simulink model "AAIver1"  (R2022a)
settings: Solver=VariableStepAuto  StartTime=0.0  StopTime=10.0  RelTol=1e-3
undefined symbols (not defined in the file): D0, D10, D11, D2, D3, D4, D8, D9, PTA0, PTA1, PTB23, PTB9, PTC16, PTC4, PTD0, PTD2
libraries: frdmk64flib x8
settings Model: Creator=Motz  LastModifiedBy=bmile

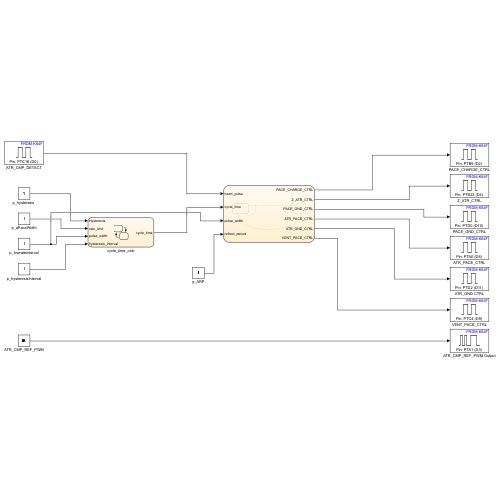
[thumbnail: Simulink's stored preview of the top-level diagram]
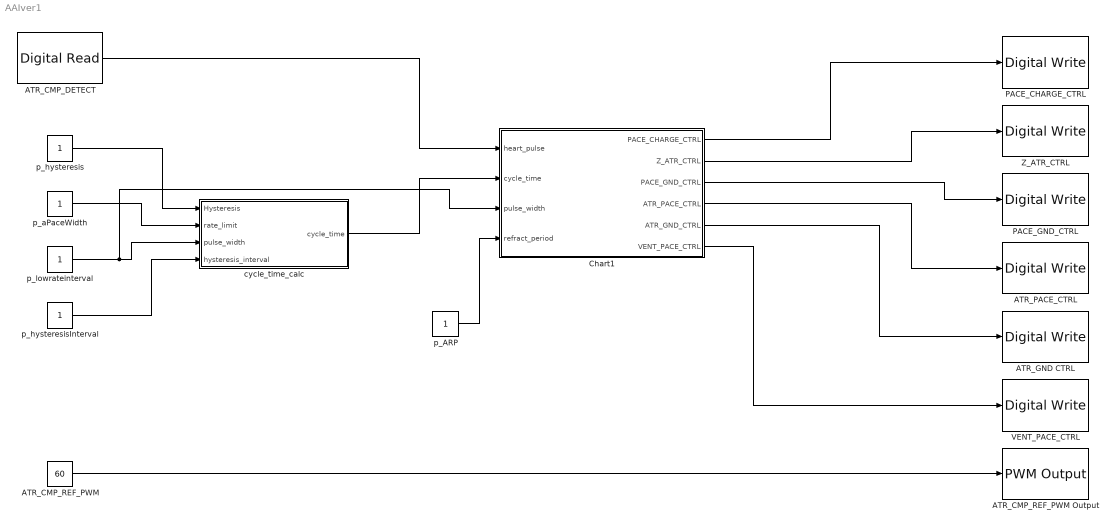
== system AAIver1 ==
  ATR_CMP_DETECT : frdmk64flib/Digital Read  Whichpin=PTC16 (D0)  SampleTime=-1
  ATR_CMP_REF_PWM : Constant  Value=60
  ATR_CMP_REF_PWM Output : frdmk64flib/PWM Output  Whichpin=PTA1 (D3)  InitialFrequency=2000  InitialDutyCycle=0
  ATR_GND CTRL : frdmk64flib/Digital Write  Whichpin=PTD2 (D11)
  ATR_PACE_CTRL : frdmk64flib/Digital Write  Whichpin=PTA0 (D8)
  Chart1 : Stateflow chart  TreatAsAtomicUnit=on
  PACE_CHARGE_CTRL : frdmk64flib/Digital Write  Whichpin=PTB9 (D2)
  PACE_GND_CTRL : frdmk64flib/Digital Write  Whichpin=PTD0 (D10)
  VENT_PACE_CTRL : frdmk64flib/Digital Write  Whichpin=PTC4 (D9)
  Z_ATR_CTRL : frdmk64flib/Digital Write  Whichpin=PTB23 (D4)
  cycle_time_calc : Stateflow chart  TreatAsAtomicUnit=on
      settings: PortSchema="{\"entries\":[{\"content\":{\"sides\":[{\"content\":{\"connectorIds\":[\"In1\",\"In2\",\"In4\",\"In3\"]},\"type\":\"ConnectorPlacement.EquallySpacedRectSide\",\"uuid\":\"0a7d0b3b-55bc-4c6a-8e46-ab8e8d3ba457\"},{\"content\":{\"connectorIds\":[\"Out1\"],\"side\":\"RIGHT\"},\"type\":\"ConnectorPlacement.EquallySpacedRectSide\",\"uuid\":\"eaa3c3bc-2449-459b-9c1e-a00ffc7b6bdb\"},{\"content\":{\"connectorIds\":[],\"side\":\"TOP\"},\"type\":\"ConnectorPlacement.EquallySpacedRectSide\",\"uuid\":\"cf212f67-e78d-4dc2-8907-6a40dfe3984c\"}]},\"type\":\"ConnectorPlacement.EquallySpacedConnector\",\"uuid\":\"bcbde97b-d1ed-422e-8255-42d4264b36d9\"}],\"packageUris\":[\"http://schema.mathworks.com/mf0/Connector/R2020b\"],\"version\":\"1.0\"}"
  p_ARP : Constant
  p_aPaceWidth : Constant
  "p_hysteresis " : Constant  OutDataTypeStr=boolean
  p_hysteresisInterval : Constant
  p_lowrateinterval : Constant
  wires:
  "p_hysteresis "/1 -> cycle_time_calc/1(Hysteresis)
  cycle_time_calc/1(cycle_time) -> Chart1/2(cycle_time)
  p_aPaceWidth/1 -> cycle_time_calc/2(rate_limit)
  p_lowrateinterval/1 -> Chart1/3(pulse_width), cycle_time_calc/4(pulse_width)
  Chart1/1(PACE_CHARGE_CTRL) -> PACE_CHARGE_CTRL/1
  Chart1/2(Z_ATR_CTRL) -> Z_ATR_CTRL/1
  Chart1/3(PACE_GND_CTRL) -> PACE_GND_CTRL/1
  Chart1/4(ATR_PACE_CTRL) -> ATR_PACE_CTRL/1
  Chart1/5(ATR_GND_CTRL) -> ATR_GND CTRL/1
  p_hysteresisInterval/1 -> cycle_time_calc/3(hysteresis_interval)
  ATR_CMP_DETECT/1 -> Chart1/1(heart_pulse)
  Chart1/6(VENT_PACE_CTRL) -> VENT_PACE_CTRL/1
  p_ARP/1 -> Chart1/4(refract_period)
  ATR_CMP_REF_PWM/1 -> ATR_CMP_REF_PWM Output/1

== stateflow chart AAIver1/cycle_time_calc ==
  data: Hysteresis input; rate_limit input; hysteresis_interval input; cycle_time output; pulse_width input

== stateflow chart AAIver1/Chart1 ==
  state Charging_Discharging
    entry:
    ATR_PACE_CTRL = false
    VENT_PACE_CTRL=false
    PACE_CHARGE_CTRL = true
    ATR_GND_CTRL = true
    PACE_GND_CTRL = true
    Z_ATR_CTRL=false
  state Pace_Heart
    entry:
    ATR_PACE_CTRL = true
    PACE_CHARGE_CTRL = false
    PACE_GND_CTRL = true
    ATR_GND_CTRL = false
  (default) -> Charging_Discharging
  Charging_Discharging -> (junction 19)
  (junction 19) -> Pace_Heart [order 1] : [~hasChanged(heart_pulse)&&after(cycle_time-pulse_width,msec)]
  (junction 19) -> Charging_Discharging [order 2] : after(refract_period,msec)
  Pace_Heart -> Charging_Discharging : after(pulse_width,msec)
  data: heart_pulse input; cycle_time input; PACE_CHARGE_CTRL output; Z_ATR_CTRL output; PACE_GND_CTRL output; ATR_PACE_CTRL output; ATR_GND_CTRL output; pulse_width input; VENT_PACE_CTRL output; refract_period input
